simulink model "BPM_HA_Variants"  (R2022b)
settings: Solver=FixedStepDiscrete  StartTime=0.0  StopTime=10.0  FixedStep=TimeSteps.ModelStep  RelTol=1e-3
settings Model: Creator=KIRTACA  LastModifiedBy=BEDNASA
settings SolverCC: AlgebraicLoopSolver=TrustRegion
settings DataIOCC: ReturnWorkspaceOutputs=off
settings DebuggingCC: UnconnectedInputMsg=warning  UnconnectedOutputMsg=warning  UnconnectedLineMsg=warning  SFMachineParentedDataDiag=warning  ArithmeticOperatorsInVariantConditions=warning
settings ModelReferenceCC: EnableRefExpFcnMdlSchedulingChecks=on
settings SFSimCC: SimUseLocalCustomCode=off  CustomCodeUndefinedFunction=UseInterfaceOnly
settings RTWCC: RTWUseLocalCustomCode=off  RTWUseSimCustomCode=on
settings CodeAppCC: StateflowObjectComments=on

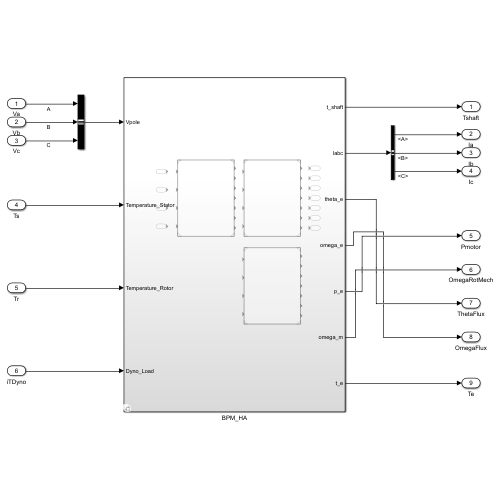
[thumbnail: Simulink's stored preview of the top-level diagram]
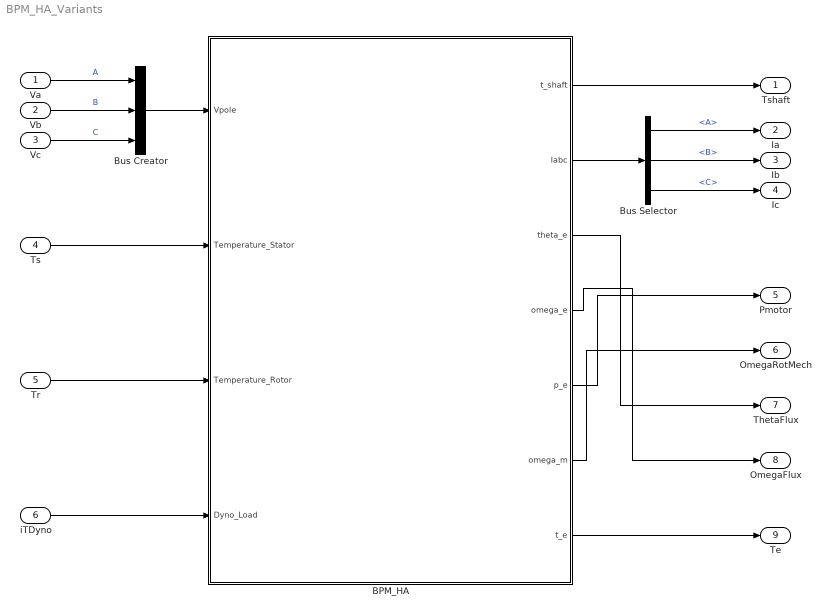
== system BPM_HA_Variants ==
  Va : Inport
  Vb : Inport  Port=2
  Vc : Inport  Port=3
  Ts : Inport  Port=4
  Tr : Inport  Port=5
  iTDyno : Inport  Port=6
  BPM_HA : Subsystem  Variant=on  VariantControl=Variant1
  Bus Creator : BusCreator  Inputs=3
  Bus Selector : BusSelector  OutputSignals=A,B,C
  Tshaft : Outport  VectorParamsAs1DForOutWhenUnconnected=off
  Ia : Outport  Port=2  VectorParamsAs1DForOutWhenUnconnected=off
  Ib : Outport  Port=3  VectorParamsAs1DForOutWhenUnconnected=off
  Ic : Outport  Port=4  VectorParamsAs1DForOutWhenUnconnected=off
  Pmotor : Outport  Port=5  VectorParamsAs1DForOutWhenUnconnected=off
  OmegaRotMech : Outport  Port=6  VectorParamsAs1DForOutWhenUnconnected=off
  ThetaFlux : Outport  Port=7  VectorParamsAs1DForOutWhenUnconnected=off
  OmegaFlux : Outport  Port=8  VectorParamsAs1DForOutWhenUnconnected=off
  Te : Outport  Port=9  VectorParamsAs1DForOutWhenUnconnected=off
  wires:
  Bus Selector/2 -> Ib/1  "<B>"
  Bus Selector/1 -> Ia/1  "<A>"
  BPM_HA/5(p_e) -> Pmotor/1
  BPM_HA/1(t_shaft) -> Tshaft/1
  BPM_HA/6(omega_m) -> OmegaRotMech/1
  BPM_HA/3(theta_e) -> ThetaFlux/1
  BPM_HA/2(Iabc) -> Bus Selector/1
  BPM_HA/4(omega_e) -> OmegaFlux/1
  Bus Selector/3 -> Ic/1  "<C>"
  BPM_HA/7(t_e) -> Te/1
  Vb/1 -> Bus Creator/2  "B"
  iTDyno/1 -> BPM_HA/4(Dyno_Load)
  Ts/1 -> BPM_HA/2(Temperature_Stator)
  Bus Creator/1 -> BPM_HA/1(Vpole)
  Vc/1 -> Bus Creator/3  "C"
  Va/1 -> Bus Creator/1  "A"
  Tr/1 -> BPM_HA/3(Temperature_Rotor)

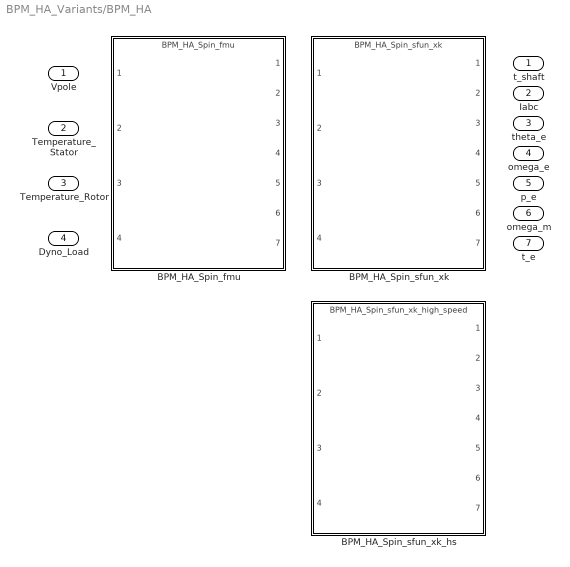
== system BPM_HA_Variants/BPM_HA ==
  Vpole : Inport  OutDataTypeStr=Bus: XabcBus
  Temperature_Stator : Inport  Port=2
  Temperature_Rotor : Inport  Port=3
  Dyno_Load : Inport  Port=4
  BPM_HA_Spin_fmu : ModelReference  ModelNameDialog=BPM_HA_Spin_fmu.slx  UsingDefaultArgumentValue=0,0,0,0,0,0,0,0,0,0,0,0,0,0,0,0,0,0,0,0,0,0,0,0,0,0,0,0,0,0,0,0,0,0,0,0,0,0,0,0,0,0,0,0,0,0,0,0,0,0,0  SimulationMode=Normal  VariantControl=Variant_Motor_Model_Executable == 1  ModelReferenceVersion=10.8  bpm_Rs_0=Motor_prm.Electrical.Rs_0  bpm_Ld_0=Motor_prm.Electrical.Ld_0  bpm_Lq_0=Motor_prm.Electrical.Lq_0  bpm_PM_flux_h1_0=Motor_prm.Electrical.PM_flux_h1_0  bpm_NPP=Motor_prm.Electrical.NPP  bpm_Jrotor=Motor_prm.Mechanical.Jrotor  bpm_B=Motor_prm.Mechanical.B  bpm_TR=Motor_prm.Mechanical.TR  bpm_Temp_stator_0=Motor_prm.Thermal.Temp_stator_0  bpm_Temp_rotor_0=Motor_prm.Thermal.Temp_rotor_0  bpm_Rs_stator_alpha=Motor_prm.Thermal.Rs_alpha  bpm_PM_rotor_alpha=Motor_prm.Thermal.PM_alpha  bpm_Ls_sat_flag=1  bpm_Loss_flag=Motor_prm.Power_Loss.Flag  bpm_Loss_th=10  bpm_Rsa_aux=0  bpm_Rsb_aux=0  bpm_Rsc_aux=0  Mech_HAs_J_drum=Mechanical.JDrum  Mech_HAs_damp=Mechanical.damp  Mech_HAs_m_unb=Mechanical.m_unb  Mech_HAs_r_unb=Mechanical.r_unb  Mech_HAs_TR=Motor_prm.Mechanical.TR  Mech_HAs_CF=0  Mech_VAa_water_vol=0  Mech_VAa_imp_dens=0  Mech_VAa_gear_ratio=0  Mech_VAa_clothes_mass=0  Mech_VAa_belt_ratio=0  Mech_VAa_basket_dia=0  Mech_VAa_basket_dens=0  Mech_VAa_J_basket=0  Mech_VAa_J_impeller=0  Mech_VAs_m_u=0  Mech_VAs_m_t=0  Mech_VAs_m_d=0  Mech_VAs_m_b1=0  Mech_VAs_m_b2=0  Mech_VAs_e=0  Mech_VAs_d=0  Mech_VAs_belt_rat=0  Mech_VAs_T_f=0  Mech_VAs_K=0  Mech_VAs_I_zt=0  Mech_VAs_D_r=0  SimulationMode=Normal
  BPM_HA_Spin_sfun_xk : ModelReference  ModelNameDialog=BPM_HA_Spin_sfun_xk  UsingDefaultArgumentValue=0,0,0,0,0,0,0,0,0,0,0,0,0,0,0,0,0,0,0,0,0,0,0,0,0,0,0,0,0,0,0,0,0,0,0,0,0,0,0,0,0,0,0,0,0,0,0,0,0,0,0  SimulationMode=Normal  VariantControl=Variant_Motor_Model_Executable == 2  ModelReferenceVersion=10.9  bpm_Rs_0=Motor_prm.Electrical.Rs_0  bpm_Ld_0=Motor_prm.Electrical.Ld_0  bpm_Lq_0=Motor_prm.Electrical.Lq_0  bpm_PM_flux_h1_0=Motor_prm.Electrical.PM_flux_h1_0  bpm_NPP=Motor_prm.Electrical.NPP  bpm_Jrotor=Motor_prm.Mechanical.Jrotor  bpm_B=Motor_prm.Mechanical.B  bpm_TR=Motor_prm.Mechanical.TR  bpm_Temp_stator_0=Motor_prm.Thermal.Temp_stator_0  bpm_Temp_rotor_0=Motor_prm.Thermal.Temp_rotor_0  bpm_Rs_stator_alpha=Motor_prm.Thermal.Rs_alpha  bpm_PM_rotor_alpha=Motor_prm.Thermal.PM_alpha  bpm_Ls_sat_flag=1  bpm_Loss_flag=Motor_prm.Power_Loss.Flag  bpm_Loss_th=10  bpm_Rsa_aux=0  bpm_Rsb_aux=0  bpm_Rsc_aux=0  Mech_HAs_J_drum=Mechanical.JDrum  Mech_HAs_damp=Mechanical.damp  Mech_HAs_m_unb=Mechanical.m_unb  Mech_HAs_r_unb=Mechanical.r_unb  Mech_HAs_TR=Motor_prm.Mechanical.TR  Mech_HAs_CF=0  Mech_VAa_water_vol=0  Mech_VAa_imp_dens=0  Mech_VAa_gear_ratio=0  Mech_VAa_clothes_mass=0  Mech_VAa_belt_ratio=0  Mech_VAa_basket_dia=0  Mech_VAa_basket_dens=0  Mech_VAa_J_basket=0  Mech_VAa_J_impeller=0  Mech_VAs_m_u=0  Mech_VAs_m_t=0  Mech_VAs_m_d=0  Mech_VAs_m_b1=0  Mech_VAs_m_b2=0  Mech_VAs_e=0  Mech_VAs_d=0  Mech_VAs_belt_rat=0  Mech_VAs_T_f=0  Mech_VAs_K=0  Mech_VAs_I_zt=0  Mech_VAs_D_r=0  SimulationMode=Normal
  BPM_HA_Spin_sfun_xk_hs : ModelReference  ModelNameDialog=BPM_HA_Spin_sfun_xk_high_speed.slx  UsingDefaultArgumentValue=0,0,0,0,0,0,0,0,0,0,0,0,0,0,0,0,0,0,0,0,0,0,0,0,0,0,0,0,0,0,0,0,0,0,0,0,0,0,0,0,0,0,0,0,0,0,0,0,0,0,0  SimulationMode=Normal  VariantControl=Variant_Motor_Model_Executable == 21  ModelReferenceVersion=10.10  bpm_Rs_0=Motor_prm.Electrical.Rs_0  bpm_Ld_0=Motor_prm.Electrical.Ld_0  bpm_Lq_0=Motor_prm.Electrical.Lq_0  bpm_PM_flux_h1_0=Motor_prm.Electrical.PM_flux_h1_0  bpm_NPP=Motor_prm.Electrical.NPP  bpm_Jrotor=Motor_prm.Mechanical.Jrotor  bpm_B=Motor_prm.Mechanical.B  bpm_TR=Motor_prm.Mechanical.TR  bpm_Temp_stator_0=Motor_prm.Thermal.Temp_stator_0  bpm_Temp_rotor_0=Motor_prm.Thermal.Temp_rotor_0  bpm_Rs_stator_alpha=Motor_prm.Thermal.Rs_alpha  bpm_PM_rotor_alpha=Motor_prm.Thermal.PM_alpha  bpm_Ls_sat_flag=1  bpm_Loss_flag=Motor_prm.Power_Loss.Flag  bpm_Loss_th=10  bpm_Rsa_aux=0  bpm_Rsb_aux=0  bpm_Rsc_aux=0  Mech_HAs_J_drum=Mechanical.JDrum  Mech_HAs_damp=Mechanical.damp  Mech_HAs_m_unb=Mechanical.m_unb  Mech_HAs_r_unb=Mechanical.r_unb  Mech_HAs_TR=Motor_prm.Mechanical.TR  Mech_HAs_CF=0  Mech_VAa_water_vol=0  Mech_VAa_imp_dens=0  Mech_VAa_gear_ratio=0  Mech_VAa_clothes_mass=0  Mech_VAa_belt_ratio=0  Mech_VAa_basket_dia=0  Mech_VAa_basket_dens=0  Mech_VAa_J_basket=0  Mech_VAa_J_impeller=0  Mech_VAs_m_u=0  Mech_VAs_m_t=0  Mech_VAs_m_d=0  Mech_VAs_m_b1=0  Mech_VAs_m_b2=0  Mech_VAs_e=0  Mech_VAs_d=0  Mech_VAs_belt_rat=0  Mech_VAs_T_f=0  Mech_VAs_K=0  Mech_VAs_I_zt=0  Mech_VAs_D_r=0  SimulationMode=Normal
  t_shaft : Outport  VectorParamsAs1DForOutWhenUnconnected=off
  Iabc : Outport  Port=2  OutDataTypeStr=Bus: XabcBus  VectorParamsAs1DForOutWhenUnconnected=off
  theta_e : Outport  Port=3  VectorParamsAs1DForOutWhenUnconnected=off
  omega_e : Outport  Port=4  VectorParamsAs1DForOutWhenUnconnected=off
  p_e : Outport  Port=5  VectorParamsAs1DForOutWhenUnconnected=off
  omega_m : Outport  Port=6  VectorParamsAs1DForOutWhenUnconnected=off
  t_e : Outport  Port=7  VectorParamsAs1DForOutWhenUnconnected=off
